simulink library "qss_tb_library"  (Simulink 8.3)
settings: Solver=ode45  SolverMode=SingleTasking  StartTime=0.0  StopTime=10.0  RelTol=1e-3
undefined symbols (not defined in the file): c_BT_E1, c_BT_E2, c_BT_E3, c_BT_E4, c_BT_L1, c_BT_L2, c_BT_L3, c_BT_L4, cc_done, delta_h_C_air, dw_GG_c, eta_EG_map, eta_EM_map, g, h, H_o_m, H_u, I_BT_max, i_FC_in, i_FC_max, k1, k2, k3, k4, k_cs, M_air, manual_gearbox, P_CVT_opt, Q_BT_0, Q_BT_IC, Q_BT_min, Q_SC_IC, rho, rho_f, t_c, T_CE_max, T_EG_c, T_EG_max, T_EM_max, U_BT_0, V_CE_map, V_FC_out, w_CE_max, w_CE_upper, w_CVT_opt, w_EG_row, w_EG_upper, w_EM_row, w_EM_upper, w_GG_c
(part 2 of 2)

== system qss_tb_library/Energy Converter/Combustion Engine (consumption map)/Detect overload and overspeed ==
  w_CE : Inport
  T_CE : Inport  Port=2
  Abs : Abs  SaturateOnIntegerOverflow=on
  Constant : Constant  Value=w_CE_upper
  Maximum torque : Lookup  InputValues=w_CE_max  Table=T_CE_max  SaturateOnIntegerOverflow=on
  Saturation : Saturate  UpperLimit=0  LowerLimit=-inf
  Saturation1 : Saturate  UpperLimit=0  LowerLimit=-inf
  Stop Simulation : Stop
  Stop Simulation1 : Stop
  Sum : Sum  Inputs=+-  SaturateOnIntegerOverflow=on  InputSameDT=on  OutDataTypeStr=Inherit: Same as first input
  Sum1 : Sum  Inputs=+-  SaturateOnIntegerOverflow=on  InputSameDT=on  OutDataTypeStr=Inherit: Same as first input
  wires:
  Sum/1 -> Saturation/1
  w_CE/1 -> Maximum torque/1, Sum1/2
  T_CE/1 -> Abs/1
  Maximum torque/1 -> Sum/1
  Abs/1 -> Sum/2
  Saturation/1 -> Stop Simulation/1
  Constant/1 -> Sum1/1
  Sum1/1 -> Saturation1/1
  Saturation1/1 -> Stop Simulation1/1

== system qss_tb_library/Energy Converter/Electric Generator/Detect overload and overspeed ==
  w_EG : Inport
  T_EG : Inport  Port=2
  Abs : Abs  SaturateOnIntegerOverflow=on
  Constant : Constant  Value=w_EG_upper
  Maximum torque : Lookup  InputValues=w_EG_row  Table=T_EG_max  SaturateOnIntegerOverflow=on
  Saturation : Saturate  UpperLimit=0  LowerLimit=-inf
  Saturation1 : Saturate  UpperLimit=0  LowerLimit=-inf
  Stop Simulation : Stop
  Stop Simulation1 : Stop
  Sum : Sum  Inputs=+-  SaturateOnIntegerOverflow=on  InputSameDT=on  OutDataTypeStr=Inherit: Same as first input
  Sum1 : Sum  Inputs=+-  SaturateOnIntegerOverflow=on  InputSameDT=on  OutDataTypeStr=Inherit: Same as first input
  wires:
  Sum/1 -> Saturation/1
  w_EG/1 -> Maximum torque/1, Sum1/2
  T_EG/1 -> Abs/1
  Maximum torque/1 -> Sum/1
  Abs/1 -> Sum/2
  Saturation/1 -> Stop Simulation/1
  Constant/1 -> Sum1/1
  Sum1/1 -> Saturation1/1
  Saturation1/1 -> Stop Simulation1/1

== system qss_tb_library/Energy Converter/Electric Motor/Detect overload and overspeed ==
  w_EM : Inport
  T_EM : Inport  Port=2
  Abs : Abs  SaturateOnIntegerOverflow=on
  Constant : Constant  Value=w_EM_upper
  Maximum torque : Lookup  InputValues=w_EM_row  Table=T_EM_max  SaturateOnIntegerOverflow=on
  Saturation : Saturate  UpperLimit=0  LowerLimit=-inf
  Saturation1 : Saturate  UpperLimit=0  LowerLimit=-inf
  Stop Simulation : Stop
  Stop Simulation1 : Stop
  Sum : Sum  Inputs=+-  SaturateOnIntegerOverflow=on  InputSameDT=on  OutDataTypeStr=Inherit: Same as first input
  Sum1 : Sum  Inputs=+-  SaturateOnIntegerOverflow=on  InputSameDT=on  OutDataTypeStr=Inherit: Same as first input
  wires:
  Saturation1/1 -> Stop Simulation1/1
  Sum1/1 -> Saturation1/1
  Constant/1 -> Sum1/1
  Saturation/1 -> Stop Simulation/1
  Abs/1 -> Sum/2
  Maximum torque/1 -> Sum/1
  T_EM/1 -> Abs/1
  w_EM/1 -> Sum1/2, Maximum torque/1
  Sum/1 -> Saturation/1

== system qss_tb_library/Energy Converter/Fuel Cell/Compressor with E-motor ==
  note: Air mass flow
  P_FC : Inport
  1/2 O2 for 1 H2 : Gain  Gain=1/2  SaturateOnIntegerOverflow=on  OutDataTypeStr=Inherit: Same as input  ParamDataTypeStr=Inherit: Same as input
  Air enthalpy : Gain  Gain=delta_h_C_air  SaturateOnIntegerOverflow=on  OutDataTypeStr=Inherit: Same as input  ParamDataTypeStr=Inherit: Same as input
  Air to fuel ratio : Gain  Gain=l_air  SaturateOnIntegerOverflow=on  OutDataTypeStr=Inherit: Same as input  ParamDataTypeStr=Inherit: Same as input
  E-motor efficiency : Gain  Gain=1/eta_EM_C  SaturateOnIntegerOverflow=on  OutDataTypeStr=Inherit: Same as input  ParamDataTypeStr=Inherit: Same as input
  Inverse O2  fraction : Gain  Gain=100/21  SaturateOnIntegerOverflow=on  OutDataTypeStr=Inherit: Same as input  ParamDataTypeStr=Inherit: Same as input
  Lower heating value : Gain  Gain=1/H_o_m  SaturateOnIntegerOverflow=on  OutDataTypeStr=Inherit: Same as input  ParamDataTypeStr=Inherit: Same as input
  Molecular weight : Gain  Gain=M_air  SaturateOnIntegerOverflow=on  OutDataTypeStr=Inherit: Same as input  ParamDataTypeStr=Inherit: Same as input
  To Workspace4 : ToWorkspace  VariableName=P_EM_C  SampleTime=1
  Unit Delay : UnitDelay  SampleTime=h
  P_EM_C : Outport  InitialOutput=0
  wires:
  Air enthalpy/1 -> E-motor efficiency/1
  Air to fuel ratio/1 -> Air enthalpy/1
  Unit Delay/1 -> Lower heating value/1
  Molecular weight/1 -> Air to fuel ratio/1
  Lower heating value/1 -> 1/2 O2 for 1 H2/1
  1/2 O2 for 1 H2/1 -> Inverse O2  fraction/1
  Inverse O2  fraction/1 -> Molecular weight/1
  E-motor efficiency/1 -> P_EM_C/1, To Workspace4/1
  P_FC/1 -> Unit Delay/1

== system qss_tb_library/Energy Converter/Fuel Cell/Supervision of current density ==
  "   i_FC" : Inport
  Constant6 : Constant  Value=i_FC_max
  Saturation1 : Saturate  UpperLimit=0  LowerLimit=-inf
  Stop Simulation : Stop
  Sum1 : Sum  Inputs=+-  SaturateOnIntegerOverflow=on  InputSameDT=on  OutDataTypeStr=Inherit: Same as first input
  wires:
  "   i_FC"/1 -> Sum1/2
  Constant6/1 -> Sum1/1
  Sum1/1 -> Saturation1/1
  Saturation1/1 -> Stop Simulation/1

== system qss_tb_library/Energy Source/Tank/Integration ==
  P_fuel : Inport
  Constant : Constant  Value=1/H_u
  Fuel consumption : UnitDelay  SampleTime=h
  Gain3 : Gain  Gain=.5*h  SaturateOnIntegerOverflow=on  OutDataTypeStr=Inherit: Same as input  ParamDataTypeStr=Inherit: Same as input
  Product2 : Product  SaturateOnIntegerOverflow=on  RndMeth=Zero  InputSameDT=on  OutDataTypeStr=Inherit: Same as first input
  Sum1 : Sum  SaturateOnIntegerOverflow=on  InputSameDT=on  OutDataTypeStr=Inherit: Same as first input
  Sum4 : Sum  SaturateOnIntegerOverflow=on  InputSameDT=on  OutDataTypeStr=Inherit: Same as first input
  To Workspace1 : ToWorkspace  VariableName=m_dot_fuel  SampleTime=-1
  To Workspace2 : ToWorkspace  VariableName=m_fuel  SampleTime=-1
  Unit Delay3 : UnitDelay  SampleTime=h
  m_fuel : Outport  InitialOutput=0
  wires:
  Constant/1 -> Product2/1
  Gain3/1 -> Product2/2
  P_fuel/1 -> Sum1/1, Unit Delay3/1
  Unit Delay3/1 -> Sum1/2
  Sum1/1 -> Gain3/1
  Fuel consumption/1 -> m_fuel/1, Sum4/1, To Workspace2/1
  Sum4/1 -> Fuel consumption/1
  Product2/1 -> Sum4/2, To Workspace1/1

== system qss_tb_library/Gear System/Continuously Variable Transmission/Power flow ==
  w_wheel : Inport
  T_wheel : Inport  Port=2
  j_CVT : Inport  Port=3
  "Engine -> Wheel" : Subsystem
  "Pwer Wheel -> Engine" : Subsystem
  Switch1 : Switch  SaturateOnIntegerOverflow=on  InputSameDT=on
  T_CVT : Outport  InitialOutput=0
  wires:
  "Pwer Wheel -> Engine"/1(T_CVT-) -> Switch1/3
  "Engine -> Wheel"/1(T_CVT+) -> Switch1/1
  Switch1/1 -> T_CVT/1
  j_CVT/1 -> "Engine -> Wheel"/3(j_CVT), "Pwer Wheel -> Engine"/3(j_CVT)
  w_wheel/1 -> "Pwer Wheel -> Engine"/1(w_wheel), "Engine -> Wheel"/1(w_wheel)
  T_wheel/1 -> "Pwer Wheel -> Engine"/2(T_wheel), "Engine -> Wheel"/2(T_wheel), Switch1/2

== system qss_tb_library/Gear System/Manual Gear Box/Power flow ==
  w_wheel : Inport
  T_wheel : Inport  Port=2
  gear : Inport  Port=3
  "Engine -> Wheel" : Subsystem
  Switch1 : Switch  SaturateOnIntegerOverflow=on  InputSameDT=on
  "Wheel -> Engine" : Subsystem
  T_MGB : Outport  InitialOutput=0
  wires:
  w_wheel/1 -> "Wheel -> Engine"/1(w_wheel), "Engine -> Wheel"/1(w_wheel)
  gear/1 -> "Wheel -> Engine"/3(gear), "Engine -> Wheel"/3(gear)
  "Wheel -> Engine"/1(T_MGB-) -> Switch1/3
  T_wheel/1 -> "Wheel -> Engine"/2(T_wheel), "Engine -> Wheel"/2(T_wheel), Switch1/2
  "Engine -> Wheel"/1(T_MGB+) -> Switch1/1
  Switch1/1 -> T_MGB/1

== system qss_tb_library/Gear System/Simple Transmission/Power flow ==
  w_wheel : Inport
  T_wheel : Inport  Port=2
  gear_ratio : Inport  Port=3
  "Energy Engine -> Wheel" : Subsystem
  "Energy Wheel -> Engine" : Subsystem
  Switch1 : Switch  SaturateOnIntegerOverflow=on  InputSameDT=on
  T_trans : Outport  InitialOutput=0
  wires:
  w_wheel/1 -> "Energy Wheel -> Engine"/1(w_wheel), "Energy Engine -> Wheel"/1(w_wheel)
  gear_ratio/1 -> "Energy Wheel -> Engine"/3(gear_ratio), "Energy Engine -> Wheel"/3(gear_ratio)
  "Energy Wheel -> Engine"/1(T_trans-) -> Switch1/3
  T_wheel/1 -> "Energy Wheel -> Engine"/2(T_wheel), "Energy Engine -> Wheel"/2(T_wheel), Switch1/2
  "Energy Engine -> Wheel"/1(T_trans+) -> Switch1/1
  Switch1/1 -> T_trans/1

== system qss_tb_library/Vehicle/Vehicle/Aerodynamic resistance ==
  v : Inport
  Aerodynamic resistance : Fcn  Expr=0.5*rho*cw*A_f*u^2
  To Workspace10 : ToWorkspace  VariableName=F_aero  SampleTime=-1
  F_aero : Outport  InitialOutput=0
  wires:
  v/1 -> Aerodynamic resistance/1
  Aerodynamic resistance/1 -> F_aero/1, To Workspace10/1

== system qss_tb_library/Vehicle/Vehicle/Average speed ==
  v : Inport
  Gain5 : Gain  Gain=0.5  SaturateOnIntegerOverflow=on  OutDataTypeStr=Inherit: Same as input  ParamDataTypeStr=Inherit: Same as input
  Sum2 : Sum  SaturateOnIntegerOverflow=on  InputSameDT=on  OutDataTypeStr=Inherit: Same as first input
  Unit Delay : UnitDelay  SampleTime=h
  v_a : Outport  InitialOutput=0
  wires:
  Unit Delay/1 -> Sum2/2
  Sum2/1 -> Gain5/1
  Gain5/1 -> v_a/1
  v/1 -> Sum2/1, Unit Delay/1

== system qss_tb_library/Vehicle/Vehicle/Inertia ==
  d_v : Inport
  Inertia : Fcn  Expr=m_f*(1+mt2m_f)*u/h
  To Workspace10 : ToWorkspace  VariableName=F_iner  SampleTime=-1
  F_iner : Outport  InitialOutput=0
  wires:
  Inertia/1 -> F_iner/1, To Workspace10/1
  d_v/1 -> Inertia/1

== system qss_tb_library/Vehicle/Vehicle/Rolling resistance ==
  v : Inport
  Rolling resistance : Constant  Value=m_f*g*mu
  Switch : Switch  Criteria=u2 > Threshold  Threshold=eps
  To Workspace2 : ToWorkspace  VariableName=F_roll  SampleTime=-1
  standstill : Constant  Value=0
  F_roll : Outport
  wires:
  Switch/1 -> To Workspace2/1, F_roll/1
  v/1 -> Switch/2
  standstill/1 -> Switch/3
  Rolling resistance/1 -> Switch/1

== system qss_tb_library/Controller/Battery Controller/Geno-Group On/Clock ==
  Constant : Constant
  Sum : Sum  Inputs=+-  SaturateOnIntegerOverflow=on  InputSameDT=on  OutDataTypeStr=Inherit: Same as first input
  Unit Delay : UnitDelay  SampleTime=duration
  out_1 : Outport  InitialOutput=0
  wires:
  Constant/1 -> Sum/1
  Sum/1 -> Unit Delay/1, out_1/1
  Unit Delay/1 -> Sum/2

== system qss_tb_library/Energy Buffer/Battery/Battery voltage/Charging ==
  Q_BT : Inport
  P_BT : Inport  Port=2
  Enable : EnablePort
  Constant4 : Constant  Value=Q_BT_0
  Fcn : Fcn  Expr=(c_BT_L3*u[1]+c_BT_L1+sqrt((c_BT_L3*u[1]+c_BT_L1)^2+4*(c_BT_L4*u[1]+c_BT_L2)*(-u[2])))/2
  Gain2 : Gain  Gain=1/Q_BT_0  SaturateOnIntegerOverflow=on  OutDataTypeStr=Inherit: Same as input  ParamDataTypeStr=Inherit: Same as input
  Gain4 : Gain  Gain=1/I_0  SaturateOnIntegerOverflow=on  OutDataTypeStr=Inherit: Same as input  ParamDataTypeStr=Inherit: Same as input
  Mux : Mux  Inputs=2
  Sum4 : Sum  Inputs=-+  SaturateOnIntegerOverflow=on  InputSameDT=on  OutDataTypeStr=Inherit: Same as first input
  U_BT_L : Outport  InitialOutput=0
  wires:
  Gain4/1 -> Mux/2
  Gain2/1 -> Mux/1
  Sum4/1 -> Gain2/1
  Q_BT/1 -> Sum4/1
  Constant4/1 -> Sum4/2
  P_BT/1 -> Gain4/1
  Mux/1 -> Fcn/1
  Fcn/1 -> U_BT_L/1

== system qss_tb_library/Energy Buffer/Battery/Battery voltage/Discharging ==
  note: q
  note: P/I_0
  Q_BT : Inport
  P_BT : Inport  Port=2
  Enable : EnablePort
  Constant6 : Constant  Value=Q_BT_0
  Fcn : Fcn  Expr=(c_BT_E3*u[1]+c_BT_E1+sqrt((c_BT_E3*u[1]+c_BT_E1)^2+4*(c_BT_E4*u[1]+c_BT_E2)*(-u[2])))/2
  Gain4 : Gain  Gain=1/Q_BT_0  SaturateOnIntegerOverflow=on  OutDataTypeStr=Inherit: Same as input  ParamDataTypeStr=Inherit: Same as input
  Gain5 : Gain  Gain=1/I_0  SaturateOnIntegerOverflow=on  OutDataTypeStr=Inherit: Same as input  ParamDataTypeStr=Inherit: Same as input
  Mux : Mux  Inputs=2
  Sum7 : Sum  Inputs=-+  SaturateOnIntegerOverflow=on  InputSameDT=on  OutDataTypeStr=Inherit: Same as first input
  U_BT_E : Outport  InitialOutput=0
  wires:
  Fcn/1 -> U_BT_E/1
  Sum7/1 -> Gain4/1
  Q_BT/1 -> Sum7/1
  Constant6/1 -> Sum7/2
  P_BT/1 -> Gain5/1
  Gain4/1 -> Mux/1
  Gain5/1 -> Mux/2
  Mux/1 -> Fcn/1

== system qss_tb_library/Energy Buffer/Battery/Battery voltage/Enable charging ==
  P_BT : Inport
  Gain : Gain  Gain=-1  SaturateOnIntegerOverflow=on  OutDataTypeStr=Inherit: Same as input  ParamDataTypeStr=Inherit: Same as input
  Saturation : Saturate  UpperLimit=0  LowerLimit=-inf
  Sign : Signum
  e_E : Outport  InitialOutput=0
  wires:
  P_BT/1 -> Saturation/1
  Sign/1 -> e_E/1
  Saturation/1 -> Gain/1
  Gain/1 -> Sign/1

== system qss_tb_library/Energy Buffer/Battery/Battery voltage/Enable discharging ==
  P_BT : Inport
  Saturation : Saturate  UpperLimit=inf  LowerLimit=0
  Sign : Signum
  e_E : Outport  InitialOutput=0
  wires:
  P_BT/1 -> Saturation/1
  Sign/1 -> e_E/1
  Saturation/1 -> Sign/1

== system qss_tb_library/Energy Buffer/Battery/Battery voltage/Enable idle ==
  P_BT : Inport
  Abs : Abs  SaturateOnIntegerOverflow=on
  Constant : Constant
  Sign : Signum
  Sum4 : Sum  Inputs=-+  SaturateOnIntegerOverflow=on  InputSameDT=on  OutDataTypeStr=Inherit: Same as first input
  e_Z : Outport  InitialOutput=0
  wires:
  P_BT/1 -> Sign/1
  Sign/1 -> Abs/1
  Abs/1 -> Sum4/1
  Sum4/1 -> e_Z/1
  Constant/1 -> Sum4/2

== system qss_tb_library/Energy Buffer/Battery/Battery voltage/Idle ==
  Q_BT : Inport
  Enable : EnablePort  StatesWhenEnabling=reset
  Constant : Constant  Value=c_BT_L1
  Constant6 : Constant  Value=Q_BT_0
  Gain4 : Gain  Gain=c_BT_L3/Q_BT_0  SaturateOnIntegerOverflow=on  OutDataTypeStr=Inherit: Same as input  ParamDataTypeStr=Inherit: Same as input
  Sum7 : Sum  Inputs=-+  SaturateOnIntegerOverflow=on  InputSameDT=on  OutDataTypeStr=Inherit: Same as first input
  Sum8 : Sum  SaturateOnIntegerOverflow=on  InputSameDT=on  OutDataTypeStr=Inherit: Same as first input
  U_BT_E : Outport  InitialOutput=0
  wires:
  Sum7/1 -> Gain4/1
  Q_BT/1 -> Sum7/1
  Constant6/1 -> Sum7/2
  Gain4/1 -> Sum8/1
  Constant/1 -> Sum8/2
  Sum8/1 -> U_BT_E/1

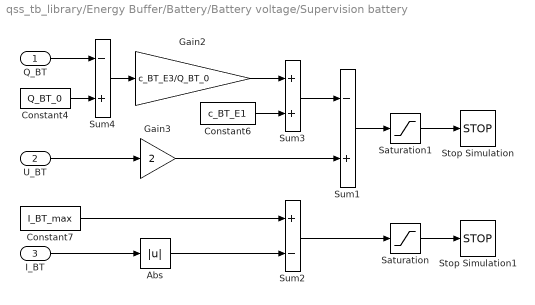
== system qss_tb_library/Energy Buffer/Battery/Battery voltage/Supervision battery ==
  Q_BT : Inport
  U_BT : Inport  Port=2
  I_BT : Inport  Port=3
  Abs : Abs  SaturateOnIntegerOverflow=on
  Constant4 : Constant  Value=Q_BT_0
  Constant6 : Constant  Value=c_BT_E1
  Constant7 : Constant  Value=I_BT_max
  Gain2 : Gain  Gain=c_BT_E3/Q_BT_0  SaturateOnIntegerOverflow=on  OutDataTypeStr=Inherit: Same as input  ParamDataTypeStr=Inherit: Same as input
  Gain3 : Gain  Gain=2  SaturateOnIntegerOverflow=on  OutDataTypeStr=Inherit: Same as input  ParamDataTypeStr=Inherit: Same as input
  Saturation : Saturate  UpperLimit=0  LowerLimit=-inf
  Saturation1 : Saturate  UpperLimit=0  LowerLimit=-inf
  Stop Simulation : Stop
  Stop Simulation1 : Stop
  Sum1 : Sum  Inputs=-+  SaturateOnIntegerOverflow=on  InputSameDT=on  OutDataTypeStr=Inherit: Same as first input
  Sum2 : Sum  Inputs=+-  SaturateOnIntegerOverflow=on  InputSameDT=on  OutDataTypeStr=Inherit: Same as first input
  Sum3 : Sum  SaturateOnIntegerOverflow=on  InputSameDT=on  OutDataTypeStr=Inherit: Same as first input
  Sum4 : Sum  Inputs=-+  SaturateOnIntegerOverflow=on  InputSameDT=on  OutDataTypeStr=Inherit: Same as first input
  wires:
  Sum3/1 -> Sum1/1
  U_BT/1 -> Gain3/1
  Gain3/1 -> Sum1/2
  Saturation/1 -> Stop Simulation1/1
  Saturation1/1 -> Stop Simulation/1
  Sum1/1 -> Saturation1/1
  Constant6/1 -> Sum3/2
  Gain2/1 -> Sum3/1
  Sum4/1 -> Gain2/1
  Q_BT/1 -> Sum4/1
  Constant4/1 -> Sum4/2
  Constant7/1 -> Sum2/1
  Sum2/1 -> Saturation/1
  I_BT/1 -> Abs/1
  Abs/1 -> Sum2/2

== system qss_tb_library/Gear System/Continuously Variable Transmission/Power flow/Engine -> Wheel ==
  w_wheel : Inport
  T_wheel : Inport  Port=2
  j_CVT : Inport  Port=3
  Constant3 : Constant  Value=P_CVT0
  Constant4 : Constant  Value=inf
  Gain : Gain  Gain=e_CVT  SaturateOnIntegerOverflow=on  OutDataTypeStr=Inherit: Same as input  ParamDataTypeStr=Inherit: Same as input
  Product4 : Product  Inputs=*/  SaturateOnIntegerOverflow=on  RndMeth=Zero  InputSameDT=on  OutDataTypeStr=Inherit: Same as first input
  Product5 : Product  Inputs=/*  SaturateOnIntegerOverflow=on  RndMeth=Zero  InputSameDT=on  OutDataTypeStr=Inherit: Same as first input
  Sum1 : Sum  SaturateOnIntegerOverflow=on  InputSameDT=on  OutDataTypeStr=Inherit: Same as first input
  Switch2 : Switch  Threshold=w_wheel_min  SaturateOnIntegerOverflow=on  InputSameDT=on
  T_CVT+ : Outport  InitialOutput=0
  wires:
  Gain/1 -> Product4/2
  Product4/1 -> T_CVT+/1
  Sum1/1 -> Product4/1
  T_wheel/1 -> Sum1/2
  Product5/1 -> Sum1/1
  w_wheel/1 -> Switch2/1, Switch2/2
  Constant4/1 -> Switch2/3
  Switch2/1 -> Product5/1
  Constant3/1 -> Product5/2
  j_CVT/1 -> Gain/1

== system qss_tb_library/Gear System/Continuously Variable Transmission/Power flow/Pwer Wheel -> Engine ==
  w_wheel : Inport
  T_wheel : Inport  Port=2
  j_CVT : Inport  Port=3
  Constant1 : Constant  Value=P_CVT0
  Constant2 : Constant  Value=inf
  Gain1 : Gain  Gain=1/e_CVT  SaturateOnIntegerOverflow=on  OutDataTypeStr=Inherit: Same as input  ParamDataTypeStr=Inherit: Same as input
  Gain2 : Gain  Gain=1/e_CVT  SaturateOnIntegerOverflow=on  OutDataTypeStr=Inherit: Same as input  ParamDataTypeStr=Inherit: Same as input
  Product2 : Product  Inputs=*/  SaturateOnIntegerOverflow=on  RndMeth=Zero  InputSameDT=on  OutDataTypeStr=Inherit: Same as first input
  Product3 : Product  Inputs=/*  SaturateOnIntegerOverflow=on  RndMeth=Zero  InputSameDT=on  OutDataTypeStr=Inherit: Same as first input
  Sum : Sum  Inputs=-+  SaturateOnIntegerOverflow=on  InputSameDT=on  OutDataTypeStr=Inherit: Same as first input
  Switch1 : Switch  Threshold=w_wheel_min  SaturateOnIntegerOverflow=on  InputSameDT=on
  T_CVT- : Outport  InitialOutput=0
  wires:
  Sum/1 -> Product2/1
  Gain1/1 -> Product3/2
  Switch1/1 -> Product3/1
  T_wheel/1 -> Sum/2
  Product3/1 -> Sum/1
  Product2/1 -> T_CVT-/1
  w_wheel/1 -> Switch1/1, Switch1/2
  Constant1/1 -> Gain1/1
  Constant2/1 -> Switch1/3
  j_CVT/1 -> Gain2/1
  Gain2/1 -> Product2/2

== system qss_tb_library/Gear System/Manual Gear Box/Power flow/Engine -> Wheel ==
  w_wheel : Inport
  T_wheel : Inport  Port=2
  gear : Inport  Port=3
  Constant1 : Constant  Value=P_GT0
  Constant2 : Constant  Value=inf
  Gain : Gain  Gain=e_GT  SaturateOnIntegerOverflow=on  OutDataTypeStr=Inherit: Same as input  ParamDataTypeStr=Inherit: Same as input
  Product2 : Product  Inputs=*/  SaturateOnIntegerOverflow=on  RndMeth=Zero  InputSameDT=on  OutDataTypeStr=Inherit: Same as first input
  Product3 : Product  Inputs=/*  SaturateOnIntegerOverflow=on  RndMeth=Zero  InputSameDT=on  OutDataTypeStr=Inherit: Same as first input
  Sum : Sum  SaturateOnIntegerOverflow=on  InputSameDT=on  OutDataTypeStr=Inherit: Same as first input
  Switch1 : Switch  Threshold=w_wheel_min  SaturateOnIntegerOverflow=on  InputSameDT=on
  T_MGB+ : Outport  InitialOutput=0
  wires:
  T_wheel/1 -> Sum/2
  Product3/1 -> Sum/1
  Gain/1 -> Product2/2
  Product2/1 -> T_MGB+/1
  Sum/1 -> Product2/1
  w_wheel/1 -> Switch1/2, Switch1/1
  Constant2/1 -> Switch1/3
  Switch1/1 -> Product3/1
  Constant1/1 -> Product3/2
  gear/1 -> Gain/1

== system qss_tb_library/Gear System/Manual Gear Box/Power flow/Wheel -> Engine ==
  w_wheel : Inport
  T_wheel : Inport  Port=2
  gear : Inport  Port=3
  Constant1 : Constant  Value=P_GT0
  Constant2 : Constant  Value=inf
  Gain1 : Gain  Gain=e_GT  SaturateOnIntegerOverflow=on  OutDataTypeStr=Inherit: Same as input  ParamDataTypeStr=Inherit: Same as input
  Gain2 : Gain  Gain=1/e_GT  SaturateOnIntegerOverflow=on  OutDataTypeStr=Inherit: Same as input  ParamDataTypeStr=Inherit: Same as input
  Product2 : Product  Inputs=*/  SaturateOnIntegerOverflow=on  RndMeth=Zero  InputSameDT=on  OutDataTypeStr=Inherit: Same as first input
  Product3 : Product  Inputs=/*  SaturateOnIntegerOverflow=on  RndMeth=Zero  InputSameDT=on  OutDataTypeStr=Inherit: Same as first input
  Sum : Sum  SaturateOnIntegerOverflow=on  InputSameDT=on  OutDataTypeStr=Inherit: Same as first input
  Switch1 : Switch  Threshold=w_wheel_min  SaturateOnIntegerOverflow=on  InputSameDT=on
  T_MGB- : Outport  InitialOutput=0
  wires:
  w_wheel/1 -> Switch1/1, Switch1/2
  gear/1 -> Gain2/1
  Constant2/1 -> Switch1/3
  Switch1/1 -> Gain1/1
  Constant1/1 -> Product3/2
  T_wheel/1 -> Sum/1
  Gain2/1 -> Product2/2
  Product2/1 -> T_MGB-/1
  Product3/1 -> Sum/2
  Sum/1 -> Product2/1
  Gain1/1 -> Product3/1

== system qss_tb_library/Gear System/Simple Transmission/Power flow/Energy Engine -> Wheel ==
  w_wheel : Inport
  T_wheel : Inport  Port=2
  gear_ratio : Inport  Port=3
  Constant1 : Constant  Value=P_GT0
  Constant2 : Constant  Value=inf
  Gain : Gain  Gain=e_GT  SaturateOnIntegerOverflow=on  OutDataTypeStr=Inherit: Same as input  ParamDataTypeStr=Inherit: Same as input
  Product2 : Product  Inputs=*/  SaturateOnIntegerOverflow=on  RndMeth=Zero  InputSameDT=on  OutDataTypeStr=Inherit: Same as first input
  Product3 : Product  Inputs=/*  SaturateOnIntegerOverflow=on  RndMeth=Zero  InputSameDT=on  OutDataTypeStr=Inherit: Same as first input
  Sum : Sum  SaturateOnIntegerOverflow=on  InputSameDT=on  OutDataTypeStr=Inherit: Same as first input
  Switch1 : Switch  Threshold=w_wheel_min  SaturateOnIntegerOverflow=on  InputSameDT=on
  T_trans+ : Outport  InitialOutput=0
  wires:
  T_wheel/1 -> Sum/2
  Product3/1 -> Sum/1
  Gain/1 -> Product2/2
  Product2/1 -> T_trans+/1
  Sum/1 -> Product2/1
  w_wheel/1 -> Switch1/2, Switch1/1
  Constant2/1 -> Switch1/3
  Switch1/1 -> Product3/1
  Constant1/1 -> Product3/2
  gear_ratio/1 -> Gain/1

== system qss_tb_library/Gear System/Simple Transmission/Power flow/Energy Wheel -> Engine ==
  w_wheel : Inport
  T_wheel : Inport  Port=2
  gear_ratio : Inport  Port=3
  Constant1 : Constant  Value=P_GT0
  Constant2 : Constant  Value=inf
  Gain1 : Gain  Gain=e_GT  SaturateOnIntegerOverflow=on  OutDataTypeStr=Inherit: Same as input  ParamDataTypeStr=Inherit: Same as input
  Gain2 : Gain  Gain=1/e_GT  SaturateOnIntegerOverflow=on  OutDataTypeStr=Inherit: Same as input  ParamDataTypeStr=Inherit: Same as input
  Product2 : Product  Inputs=*/  SaturateOnIntegerOverflow=on  RndMeth=Zero  InputSameDT=on  OutDataTypeStr=Inherit: Same as first input
  Product3 : Product  Inputs=/*  SaturateOnIntegerOverflow=on  RndMeth=Zero  InputSameDT=on  OutDataTypeStr=Inherit: Same as first input
  Sum : Sum  SaturateOnIntegerOverflow=on  InputSameDT=on  OutDataTypeStr=Inherit: Same as first input
  Switch1 : Switch  Threshold=w_wheel_min  SaturateOnIntegerOverflow=on  InputSameDT=on
  T_trans- : Outport  InitialOutput=0
  wires:
  w_wheel/1 -> Switch1/1, Switch1/2
  gear_ratio/1 -> Gain2/1
  Constant2/1 -> Switch1/3
  Switch1/1 -> Gain1/1
  Constant1/1 -> Product3/2
  T_wheel/1 -> Sum/1
  Gain2/1 -> Product2/2
  Product2/1 -> T_trans-/1
  Product3/1 -> Sum/2
  Sum/1 -> Product2/1
  Gain1/1 -> Product3/1
